simulink model "Simu_DiscreteInt"  (R2024a)
settings: Solver=VariableStepAuto  StartTime=ti  StopTime=tf  FixedStep=dt  MaxStep=1e-1  RelTol=1e-4  AbsTol=1e-6
settings Model: Creator=perruquetti  LastModifiedBy=perruquetti
settings SolverCC: AlgebraicLoopSolver=LineSearch
settings DebuggingCC: AlgebraicLoopMsg=none  UnconnectedInputMsg=warning  UnconnectedOutputMsg=warning  UnconnectedLineMsg=warning
settings ModelReferenceCC: EnableRefExpFcnMdlSchedulingChecks=on
settings RTWCC: GPUComputeCapability=3.5  DLArmComputeVersion=19.05

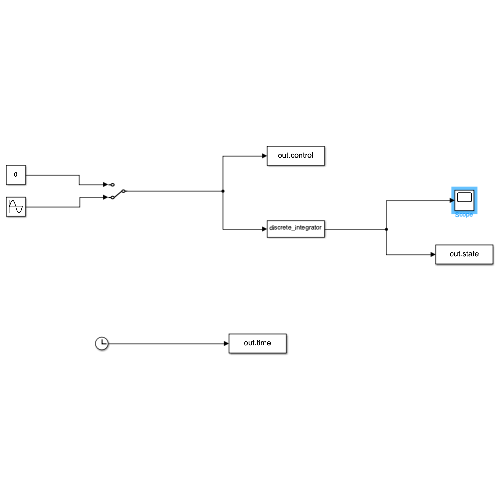
[thumbnail: Simulink's stored preview of the top-level diagram]
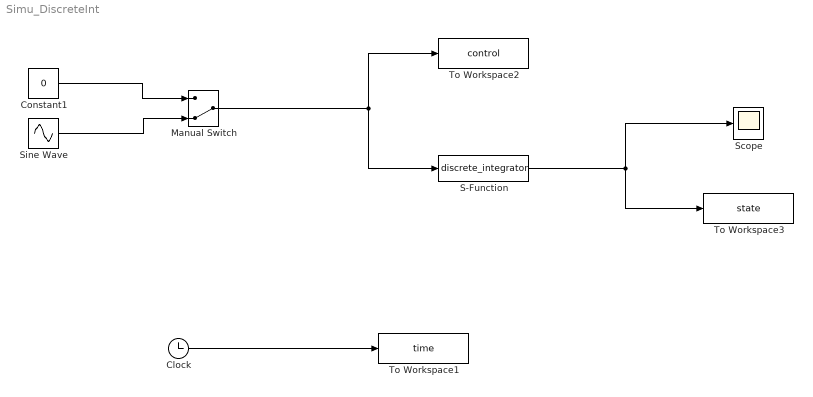
== system Simu_DiscreteInt ==
  Clock : Clock
  Constant1 : Constant  Value=0
  Manual Switch : ManualSwitch  CurrentSetting=0
  S-Function : S-Function  FunctionName=discrete_integrator  SFunctionDeploymentMode=off  EnableBusSupport=off
  Scope : Scope
  Sine Wave : Sin  SampleTime=0
  To Workspace1 : ToWorkspace  VariableName=time  SampleTime=-1
  To Workspace2 : ToWorkspace  VariableName=control  SampleTime=-1
  To Workspace3 : ToWorkspace  VariableName=state  SaveFormat=Structure With Time  SampleTime=-1
  wires:
  Clock/1 -> To Workspace1/1
  S-Function/1 -> Scope/1, To Workspace3/1
  Constant1/1 -> Manual Switch/1
  Sine Wave/1 -> Manual Switch/2
  Manual Switch/1 -> S-Function/1, To Workspace2/1
